simulink model "Universal_discrete_simulation_75"  (Simulink 7.0)
settings: Solver=FixedStepDiscrete  StartTime=0.0  StopTime=simulation_horizon  FixedStep=Ts  RelTol=1e-8  AbsTol=1e-6
values from neighbouring files (symbols this model uses):
  Cm = Cmm    [MMCE.m]
  F = zeros(n)    [MMCE.m]    (also in yalmip_lmi_reg.m = F + set(kron(Lreg,Y) + kron(Mreg,(A*Y-B*W)') + kron(Mreg',(A)
  G = zeros(n,q)    [MMCE.m]
  H = zeros(n)    [MMCE.m]
  J = zeros(n,p)    [MMCE.m]
  K = zeros(n,q)    [MMCE.m]
  L1 = L    [MMCE.m]
  L2 = zeros(p,q)    [MMCE.m]
  M = [A-lambdades(i)*eye(n) -B]    [Choice_Eigenvec_Paramvec.m]    (also in Falb_Wolovich_or_Roppenecker.m = inv(Dstar)*diag([knum]); MMCE.m = inv(G_CL),)
  n = size(A,1)    [Becker_Ostertag.m]    (also in Falb_Wolovich_or_Roppenecker.m; MMCE.m; Responses.m = size(A_CL,1); Roppenecker.m)
  p = size(B,2)    [Becker_Ostertag.m]    (also in Falb_Wolovich_or_Roppenecker.m; MMCE.m = size(Bc,2); Responses.m; Roppenecker.m)
  p_load = 1    [MMCE.m]
  p_measurements = -0.5    [MMCE.m]
  Sc = zeros(qc, q)    [MMCE.m]
  Si = zeros(q,q)    [MMCE.m]
  simulation_horizon = 15*Ts    (= 15)    [MMCE.m]
  start_p_load = 5*Ts    (= 5)    [MMCE.m]
  start_p_measurements = 10*Ts    (= 10)    [MMCE.m]
  start_reference = 0    [MMCE.m]
  Ts = 1    [MMCE.m]
  x0 = xx0    [MMCE.m]    (also in Responses.m = as above) (Y/N)? [N] --> ','s'); yalmip_lmi_reg.m = input('  Enter a real number:  '))
  yr = 1    [MMCE.m]
  z0 = 0    [MMCE.m]
undefined symbols (not defined in the file or in its folder): DiscIntNeverNeededParam, Gamma, Phi, Te
libraries: simulink x9
settings Model: Creator=Eric  LastModifiedBy=Eric  ExtModeTrigMode=oneshot  ExtModeArmWhenConnect=off
settings SolverCC: InitialStep=0.001
settings DataIOCC: LimitDataPoints=off  SignalLoggingName=sigsOut
settings OptimizationCC: BooleanDataType=off
settings DebuggingCC: SaveWithParameterizedLinksMsg=none  SignalResolutionControl=TryResolveAllWithWarning  SolverPrmCheckMsg=none  MultiTaskDSMMsg=warning  MultiTaskCondExecSysMsg=none  StrictBusMsg=None
settings HardwareCC: TargetUnknown=on
settings RTWCC: IncludeERTFirstTime=on
settings GRTTargetCC: TargetFcnLib=ansi_tfl_tmw.mat

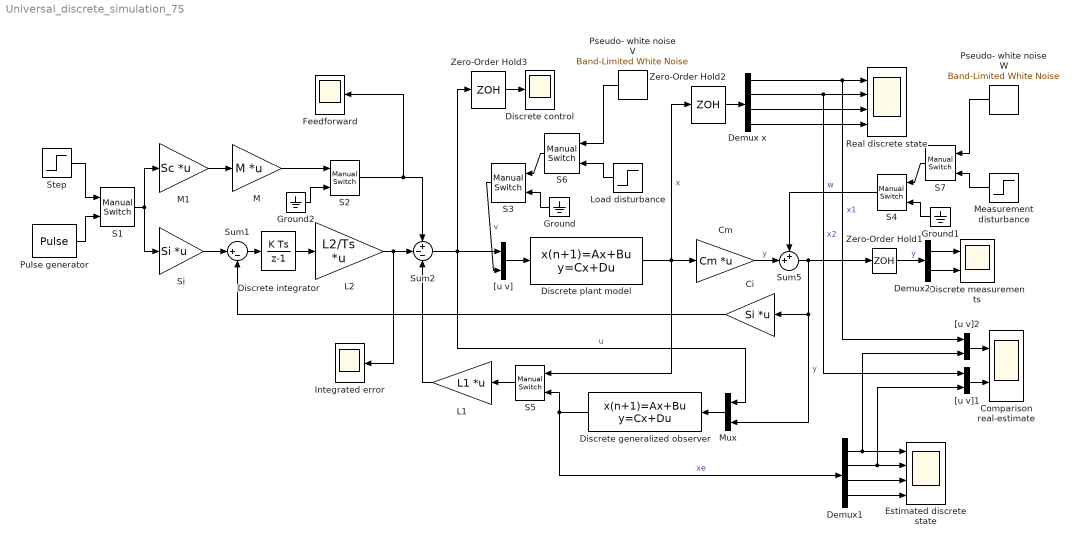
== system Universal_discrete_simulation_75 ==
  Ci : Gain  Orientation=left  Gain=Si  Multiplication=Matrix(K*u)  ParameterDataType=sfix(16)  ParameterScaling=2^0  OutDataType=sfix(16)  OutScaling=2^0  SaturateOnIntegerOverflow=on
  Cm : Gain  Gain=Cm  Multiplication=Matrix(K*u)  ParameterDataType=sfix(16)  ParameterScaling=2^0  OutDataType=sfix(16)  OutScaling=2^0  SaturateOnIntegerOverflow=on
  Comparison real-estimate : Scope  NumInputPorts=2
      settings: YMin=-0.1~-0.2  YMax=0.3~0.2  SaveName=CompareScope  MaxDataPoints=100000
  Demux x : Demux  Outputs=n
  Demux1 : Demux  Outputs=n
  Demux2 : Demux  Outputs=q
  Discrete control : Scope
      settings: YMin=-0.2  YMax=1  SaveName=ControlScope  MaxDataPoints=100000
  Discrete integrator : DiscreteIntegrator  SampleTime=Ts  OutDataType=sfix(16)  OutScaling=2^0  ICPrevOutput=DiscIntNeverNeededParam  ICPrevScaledInput=DiscIntNeverNeededParam
  Discrete measurements : Scope  NumInputPorts=2
      settings: YMin=0~-5  YMax=2.5~5  SaveName=MeasurementScope  MaxDataPoints=100000
  Discrete generalized observer : DiscreteStateSpace  Orientation=left  A=F  B=[J G]  C=H  D="[zeros(n,p)  K]"  X0=[z0]  SampleTime=Ts
  Discrete plant model : DiscreteStateSpace  A=Phi  B=[Gamma E]  C=eye(n)  D=zeros(n,p+size(E,2))  X0=[x0]  SampleTime=Ts
  Estimated discrete state : Scope  NumInputPorts=4
      settings: YMin=-0.1~-0.2~-5~-5  YMax=0.3~0.2~5~5  SaveName=EstimateScope  MaxDataPoints=200000
  Feedforward : Scope
      settings: YMin=-2  YMax=4  SaveName=ScopeData3  MaxDataPoints=100000
  Ground : Ground  Orientation=left
  Ground1 : Ground  Orientation=left
  Ground2 : Ground
  Integrated error : Scope
      settings: YMin=-2  YMax=0  MaxDataPoints=100000
  L1 : Gain  Orientation=left  Gain=L1  Multiplication=Matrix(K*u)  ParameterDataType=sfix(16)  ParameterScaling=2^0  OutDataType=sfix(16)  OutScaling=2^0  SaturateOnIntegerOverflow=on
  L2 : Gain  Gain=L2/Ts  Multiplication=Matrix(K*u)  ParameterDataType=sfix(16)  ParameterScaling=2^0  OutDataType=sfix(16)  OutScaling=2^0  SaturateOnIntegerOverflow=on
  Load disturbance : Step  Orientation=left  Time=start_p_load  Before=[0]  After=p_load*Ts  SampleTime=0
  M : Gain  Gain=M  Multiplication=Matrix(K*u)  ParameterDataType=sfix(16)  ParameterScaling=2^0  OutDataType=sfix(16)  OutScaling=2^0  SaturateOnIntegerOverflow=on
  M1 : Gain  Gain=Sc  Multiplication=Matrix(K*u)  ParameterDataType=sfix(16)  ParameterScaling=2^0  OutDataType=sfix(16)  OutScaling=2^0  SaturateOnIntegerOverflow=on
  Measurement disturbance : Step  Orientation=left  Time=start_p_measurements  Before=[0]  After=p_measurements  SampleTime=0
  Mux : Mux  Orientation=left  Inputs=2
  Pseudo- white noise V : simulink/Sources/Band-Limited White Noise  Orientation=left  SystemSampleTime=-1  Cov=eqn_pwr  Ts=Ts  seed=eqn_seed
  Pseudo- white noise W : simulink/Sources/Band-Limited White Noise  Orientation=left  SystemSampleTime=-1  Cov=meas_pwr  Ts=Ts  seed=meas_seed
  Pulse generator : DiscretePulseGenerator  PulseType=Time based  Amplitude=yr  Period=simulation_horizon/2  PulseWidth=50  SampleTime=Te
  Real discrete state : Scope  NumInputPorts=4
      settings: YMin=-0.1~-0.2~-5~-5  YMax=0.3~0.2~5~5  SaveName=StateScope  MaxDataPoints=100000
  S1 : simulink/Signal Routing/Manual Switch  SystemSampleTime=-1  sw=1  action=0  varsize=off
  S2 : simulink/Signal Routing/Manual Switch  SystemSampleTime=-1  sw=1  action=0  varsize=off
  S{3..4,6..7} (4 alike) : simulink/Signal Routing/Manual Switch  Orientation=left  SystemSampleTime=-1  sw=0  action=0  varsize=off
  S5 : simulink/Signal Routing/Manual Switch  Orientation=left  SystemSampleTime=-1  sw=1  action=0  varsize=off
  Si : Gain  Gain=Si  Multiplication=Matrix(K*u)  ParameterDataType=sfix(16)  ParameterScaling=2^0  OutDataType=sfix(16)  OutScaling=2^0  SaturateOnIntegerOverflow=on
  Step : Step  Time=start_reference  Before=[0]  After=yr  SampleTime=0
  Sum1 : Sum  Inputs=|+-  OutDataType=sfix(16)  OutScaling=2^0  SaturateOnIntegerOverflow=on  InputSameDT=on
  Sum2 : Sum  Inputs=+--  OutDataType=sfix(16)  OutScaling=2^0  SaturateOnIntegerOverflow=on  InputSameDT=on
  Sum5 : Sum  Inputs=++|  OutDataType=sfix(16)  OutScaling=2^0  SaturateOnIntegerOverflow=on
  Zero-Order Hold1 : ZeroOrderHold  SampleTime=Ts
  Zero-Order Hold2 : ZeroOrderHold  SampleTime=Ts
  Zero-Order Hold3 : ZeroOrderHold  SampleTime=Ts
  "[u v]" : Mux  Inputs=2
  "[u v]1" : Mux  Inputs=2
  "[u v]2" : Mux  Inputs=2
  wires:
  Sum1/1 -> Discrete integrator/1
  Discrete integrator/1 -> L2/1
  Demux x/2 -> Real discrete state/2, "[u v]1"/1  "x2"
  Demux x/1 -> Real discrete state/1, "[u v]2"/1  "x1"
  S3/1 -> "[u v]"/2  "v"
  Ground/1 -> S3/2
  Discrete plant model/1 -> Cm/1, Zero-Order Hold2/1, S5/1  "x"
  Ground1/1 -> S4/2
  Sum2/1 -> "[u v]"/1, Mux/1, Zero-Order Hold3/1  "u"
  "[u v]"/1 -> Discrete plant model/1
  L1/1 -> Sum2/3
  S2/1 -> Sum2/1, Feedforward/1
  Ground2/1 -> S2/2
  M/1 -> S2/1
  L2/1 -> Sum2/2, Integrated error/1
  Demux x/3 -> Real discrete state/3
  Ci/1 -> Sum1/2
  Mux/1 -> Discrete generalized observer/1
  S5/1 -> L1/1
  Demux1/1 -> Estimated discrete state/1, "[u v]2"/2
  Demux1/2 -> Estimated discrete state/2, "[u v]1"/2
  Step/1 -> S1/1
  Pulse generator/1 -> S1/2
  S1/1 -> Si/1, M1/1
  Cm/1 -> Sum5/2  "y"
  Sum5/1 -> Zero-Order Hold1/1, Mux/2, Ci/1  "y"
  S4/1 -> Sum5/1  "w"
  Measurement disturbance/1 -> S7/2
  S7/1 -> S4/1
  Pseudo- white noise W/1 -> S7/1
  Discrete generalized observer/1 -> S5/2, Demux1/1  "xe"
  S6/1 -> S3/1
  Pseudo- white noise V/1 -> S6/1
  Load disturbance/1 -> S6/2
  Zero-Order Hold2/1 -> Demux x/1
  Zero-Order Hold3/1 -> Discrete control/1
  Si/1 -> Sum1/1
  M1/1 -> M/1
  Zero-Order Hold1/1 -> Demux2/1  "y"
  Demux2/1 -> Discrete measurements/1
  Demux2/2 -> Discrete measurements/2
  Demux1/3 -> Estimated discrete state/3
  Demux1/4 -> Estimated discrete state/4
  Demux x/4 -> Real discrete state/4
  "[u v]2"/1 -> Comparison real-estimate/1
  "[u v]1"/1 -> Comparison real-estimate/2
